simulink subsystem "EvPowertrainController2EM_r3"  (R2025b)
settings: Solver=VariableStepAuto  StartTime=0.0  StopTime=10.0  RelTol=1e-3
undefined symbols (not defined in the file): CtrlVcuAccelPdlBpts, CtrlVcuBattPnlty, CtrlVcuEMPnlty, CtrlVcuEMTrqSplitGrid, CtrlVcuEvChrgLmtBpt, CtrlVcuEvRegenBrkCutOff, CtrlVcuEvRegenBrkSpdBpt, CtrlVcuEvSocBpt, CtrlVcuFallRate, CtrlVcuMaxAccelG, CtrlVcuMaxDecelG, CtrlVcuPwrRatePnlty, CtrlVcuRiseRate, CtrlVcuRoadMuEst, CtrlVcuSftyFctr, CtrlVcuTracPwrErrPnlty, DriverMode, eff, EnvGrvty, PlntBrkActrBoreFrnt, PlntBrkFrntBias, PlntBrkKinFricCffFrnt, PlntBrkNumPadsFrnt, PlntBrkPadMeanRadiusFrnt, PlntBrkPrsFctr, PlntBrkRearBias, PlntDiffrntl2Eff, PlntDiffrntl2Ratio, PlntDiffrntlEff, PlntDiffrntlRatio, PlntEM1EffTbl, PlntEM1Spd, PlntEM1Trq, PlntEM1TrqEff, PlntEM2EffTbl, PlntEM2Spd, PlntEM2Trq, PlntEM2TrqEff, PlntEM3EffTbl, PlntEM3Spd, PlntEM3Trq, PlntEM3TrqEff, PlntEMWhlGearEffFL, PlntEMWhlGearEffRL, PlntEMWhlGearRatioFL, PlntEMWhlGearRatioRL, PlntTransEffSpdBpt, PlntTransEffTbl, PlntTransEffTempBpt, PlntTransEffTrqBpt, PlntTransGearNumVect, PlntTransGearRatioVect, PlntVehCGHgtAxl, PlntVehDstCGFrntAxl, PlntVehDstCGRearAxl, PlntVehMass, PlntWhlLdRadius, RegenEnd, RegenStrt, SOCInit ... (+1)
libraries: simulink x13, autolibutils x2
(part 1 of 5)
settings Model: Creator=smuckati  LastModifiedBy=smuckati
settings RTWCC: GPUComputeCapability=3.5

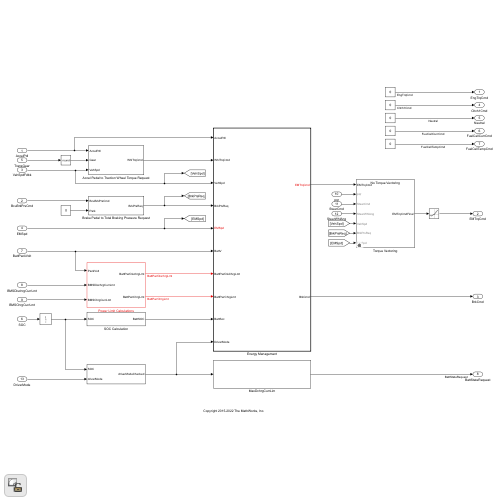
[thumbnail: Simulink's stored preview of the top-level diagram]
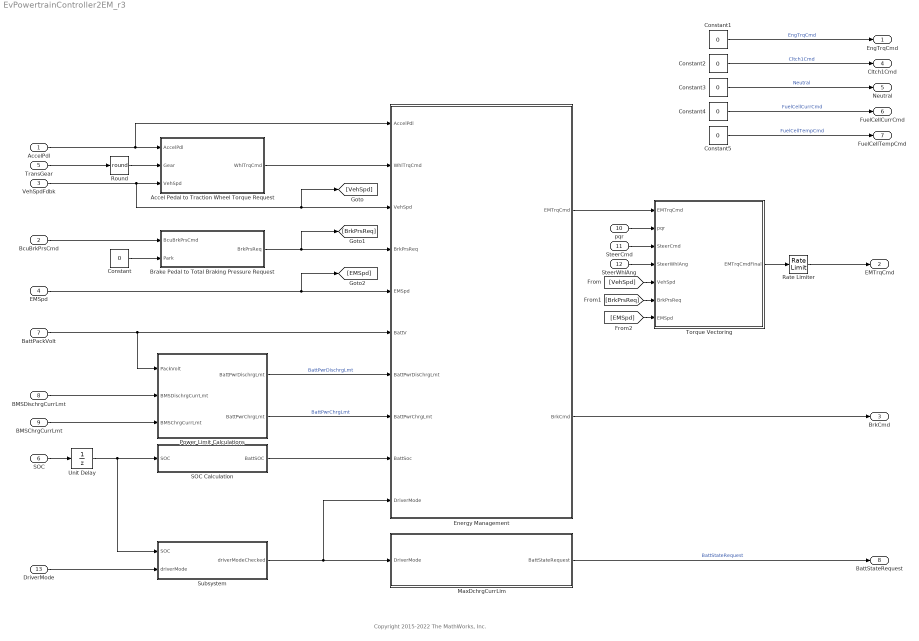
== system EvPowertrainController2EM_r3 ==
  note: Copyright 2015-2022 The MathWorks, Inc.
  AccelPdl : Inport
  BcuBrkPrsCmd : Inport  Port=2  PortDimensions=4
  VehSpdFdbk : Inport  Port=3
  EMSpd : Inport  Port=4
  TransGear : Inport  Port=5
  SOC : Inport  Port=6
  BattPackVolt : Inport  Port=7
  BMSDischrgCurrLmt : Inport  Port=8
  BMSChrgCurrLmt : Inport  Port=9
  pqr : Inport  Port=10  PortDimensions=3
  SteerCmd : Inport  Port=11
  SteerWhlAng : Inport  Port=12  PortDimensions=4
  DriverMode : Inport  Port=13
  Accel Pedal to Traction Wheel Torque Request : Subsystem  InitFcn=[~]=autosharedicon('autolibinternalvvblock',gcb,0);  VariantControl=Choice
  Brake Pedal to Total Braking Pressure Request : Subsystem  InitFcn=[~]=autosharedicon('autolibinternalvvblock',gcb,0);
  Constant{,1..5} (6 alike) : Constant  Value=0  SampleTime=-1
  Energy Management : Subsystem  LoadFcn=[~]=autosharedicon('autolibinternalvvblock',gcb,0);  TreatAsAtomicUnit=on
  MaxDchrgCurrLim : Subsystem
  Power Limit Calculations : Subsystem  InitFcn=[~]=autosharedicon('autolibinternalvvblock',gcb,0);
  Rate Limiter : RateLimiter  RisingSlewLimit=CtrlVcuRiseRate  FallingSlewLimit=CtrlVcuFallRate  SampleTimeMode=inherited
  Round : Rounding  Operator=round
  SOC Calculation : Subsystem  InitFcn=[~]=autosharedicon('autolibinternalvvblock',gcb,0);
  Subsystem : Subsystem
  Torque Vectoring : Subsystem  Variant=on  VariantControlMode=label  VariantControl=Choice  LabelModeActiveChoice=No Torque Vectoring
  Unit Delay : UnitDelay  InitialCondition=SOCInit  SampleTime=-1  HasFrameUpgradeWarning=on
  EngTrqCmd : Outport
  EMTrqCmd : Outport  Port=2
  BrkCmd : Outport  Port=3
  Cltch1Cmd : Outport  Port=4
  Neutral : Outport  Port=5
  FuelCellCurrCmd : Outport  Port=6
  FuelCellTempCmd : Outport  Port=7
  BattStateRequest : Outport  Port=8
  wires:
  Rate Limiter/1 -> EMTrqCmd/1
  AccelPdl/1 -> Accel Pedal to Traction Wheel Torque Request/1(AccelPdl), Energy Management/1(AccelPdl)
  Constant/1 -> Brake Pedal to Total Braking Pressure Request/2(Park)
  EMSpd/1 -> Energy Management/5(EMSpd), [EMSpd]
  Power Limit Calculations/2(BattPwrChrgLmt) -> Energy Management/8("BattPwrChrgLmt ")  "BattPwrChrgLmt"
  [BrkPrsReq] -> Torque Vectoring/6(BrkPrsReq)
  Accel Pedal to Traction Wheel Torque Request/1(WhlTrqCmd) -> Energy Management/2(WhlTrqCmd)
  BattPackVolt/1 -> Power Limit Calculations/1(PackVolt), Energy Management/6(BattV)
  Brake Pedal to Total Braking Pressure Request/1(BrkPrsReq) -> Energy Management/4("BrkPrsReq "), [BrkPrsReq]
  SOC Calculation/1(BattSOC) -> Energy Management/9(BattSoc)
  BcuBrkPrsCmd/1 -> Brake Pedal to Total Braking Pressure Request/1(BcuBrkPrsCmd)
  pqr/1 -> Torque Vectoring/2(pqr)
  [VehSpd] -> Torque Vectoring/5(VehSpd)
  VehSpdFdbk/1 -> Accel Pedal to Traction Wheel Torque Request/3(VehSpd), Energy Management/3(VehSpd), [VehSpd]
  SteerCmd/1 -> Torque Vectoring/3(SteerCmd)
  SteerWhlAng/1 -> Torque Vectoring/4(SteerWhlAng)
  Round/1 -> Accel Pedal to Traction Wheel Torque Request/2(Gear)
  Energy Management/2(BrkCmd) -> BrkCmd/1
  Energy Management/1(EMTrqCmd) -> Torque Vectoring/1(EMTrqCmd)
  [EMSpd] -> Torque Vectoring/7(EMSpd)
  Power Limit Calculations/1(BattPwrDischrgLmt) -> Energy Management/7(BattPwrDisChrgLmt)  "BattPwrDischrgLmt"
  Torque Vectoring/1(EMTrqCmdFinal) -> Rate Limiter/1
  Constant5/1 -> FuelCellTempCmd/1  "FuelCellTempCmd"
  MaxDchrgCurrLim/1(BattStateRequest) -> BattStateRequest/1  "BattStateRequest"
  SOC/1 -> Unit Delay/1
  TransGear/1 -> Round/1
  Constant4/1 -> FuelCellCurrCmd/1  "FuelCellCurrCmd"
  Constant2/1 -> Cltch1Cmd/1  "Cltch1Cmd"
  BMSDischrgCurrLmt/1 -> Power Limit Calculations/2(BMSDischrgCurrLmt)
  Constant1/1 -> EngTrqCmd/1  "EngTrqCmd"
  Constant3/1 -> Neutral/1  "Neutral"
  BMSChrgCurrLmt/1 -> Power Limit Calculations/3(BMSChrgCurrLmt)
  DriverMode/1 -> Subsystem/2(driverMode)
  Subsystem/1(driverModeChecked) -> MaxDchrgCurrLim/1(DriverMode), Energy Management/10(DriverMode)
  Unit Delay/1 -> SOC Calculation/1(SOC), Subsystem/1(SOC)

== system EvPowertrainController2EM_r3/Accel Pedal to Traction Wheel Torque Request ==
  note: Convert Accelerator Pedal Position to
      | Wheel Torque Command using Motor
      | Torque Speed Curves.
      |
      | Can be replaced with 2D Lookup Table
      | with AccelPdl and VehSpd as inputs and
      | Motor or Wheel Torque Command as output.
  AccelPdl : Inport
  Gear : Inport  Port=2
  VehSpd : Inport  Port=3
  EM2WhlTrq : Subsystem  Variant=on  VariantControlMode=label  VariantControl=Choice  LabelModeActiveChoice=2EM
  Product1 : Product
  WhlTrqCmd : Outport  VectorParamsAs1DForOutWhenUnconnected=off
  wires:
  EM2WhlTrq/1(WhlTrqCmd) -> Product1/2
  VehSpd/1 -> EM2WhlTrq/2(VehSpd)
  Gear/1 -> EM2WhlTrq/1(Gear)
  AccelPdl/1 -> Product1/1
  Product1/1 -> WhlTrqCmd/1

== system EvPowertrainController2EM_r3/Brake Pedal to Total Braking Pressure Request ==
  BcuBrkPrsCmd : Inport
  Park : Inport  Port=2
  Front Bias : Constant  Value=PlntBrkFrntBias
  Gain4 : Gain  Gain=PlntBrkPrsFctr
  Mux : Mux
  Product : Product
  Rear Bias : Constant  Value=PlntBrkRearBias
  Terminator : Terminator
  BrkPrsReq : Outport  VectorParamsAs1DForOutWhenUnconnected=off
  wires:
  Park/1 -> Terminator/1
  Product/1 -> Gain4/1
  Gain4/1 -> BrkPrsReq/1
  Front Bias/1 -> Mux/2, Mux/1
  Rear Bias/1 -> Mux/3, Mux/4
  Mux/1 -> Product/1
  BcuBrkPrsCmd/1 -> Product/2

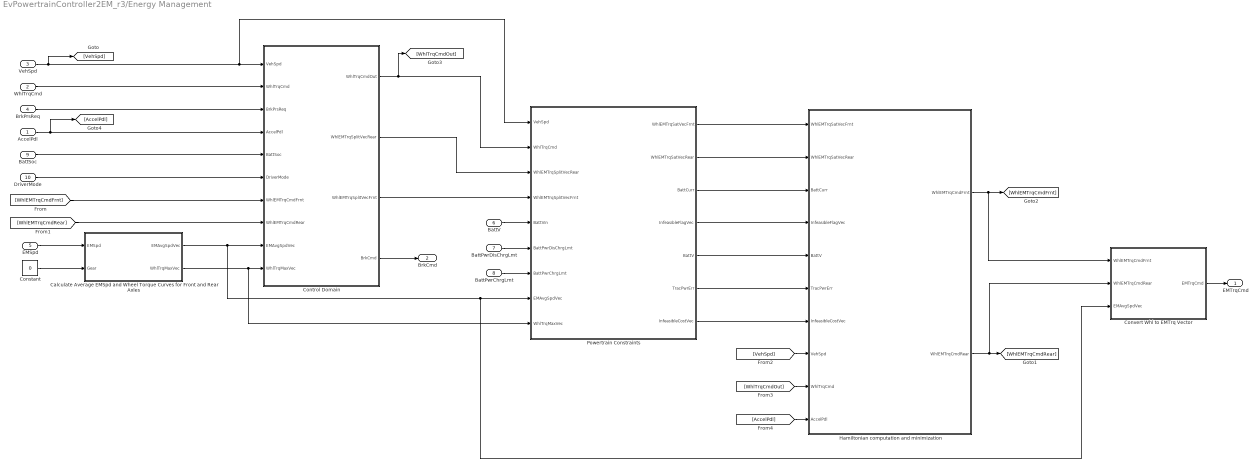
== system EvPowertrainController2EM_r3/Energy Management ==
  AccelPdl : Inport
  WhlTrqCmd : Inport  Port=2
  VehSpd : Inport  Port=3
  "BrkPrsReq " : Inport  Port=4
  EMSpd : Inport  Port=5
  BattV : Inport  Port=6
  BattPwrDisChrgLmt : Inport  Port=7
  "BattPwrChrgLmt " : Inport  Port=8
  BattSoc : Inport  Port=9
  DriverMode : Inport  Port=10
  Calculate Average EMSpd and Wheel Torque Curves for Front and Rear Axles : Subsystem  Variant=on  VariantControlMode=label  VariantControl=Choice  LabelModeActiveChoice=2EM
  Constant : Constant  Value=0  SampleTime=-1
  "Control Domain " : Subsystem  InitFcn="[~] =  autosharedeval('1');"
  Convert Whl to EMTrq Vector : Subsystem  Variant=on  VariantControlMode=label  VariantControl=Choice  LabelModeActiveChoice=2EM
  Hamiltonian computation and minimization : Subsystem  InitFcn="[~] =  autosharedeval('1');"
  "Powertrain Constraints " : Subsystem  InitFcn="[~] =  autosharedeval('1');"
  EMTrqCmd : Outport  VectorParamsAs1DForOutWhenUnconnected=off
  BrkCmd : Outport  Port=2  VectorParamsAs1DForOutWhenUnconnected=off
  wires:
  DriverMode/1 -> "Control Domain "/6(DriverMode)
  [AccelPdl] -> Hamiltonian computation and minimization/10(AccelPdl)
  [WhlTrqCmdOut] -> Hamiltonian computation and minimization/9(WhlTrqCmd)
  "Control Domain "/3(WhlEMTrqSplitVecFrnt) -> "Powertrain Constraints "/4(WhlEMTrqSplitVecFrnt)
  "Powertrain Constraints "/7(InfeasibleCostVec) -> Hamiltonian computation and minimization/7(InfeasibleCostVec)
  [VehSpd] -> Hamiltonian computation and minimization/8(VehSpd)
  "Powertrain Constraints "/2(WhlEMTrqSatVecRear) -> Hamiltonian computation and minimization/2(WhlEMTrqSatVecRear)
  "Powertrain Constraints "/1(WhlEMTrqSatVecFrnt) -> Hamiltonian computation and minimization/1(WhlEMTrqSatVecFrnt)
  Calculate Average EMSpd and Wheel Torque Curves for Front and Rear Axles/2(WhlTrqMaxVec) -> "Control Domain "/10(WhlTrqMaxVec), "Powertrain Constraints "/9(WhlTrqMaxVec)
  Constant/1 -> Calculate Average EMSpd and Wheel Torque Curves for Front and Rear Axles/2(Gear)
  [WhlEMTrqCmdRear] -> "Control Domain "/8(WhlEMTrqCmdRear)
  Convert Whl to EMTrq Vector/1(EMTrqCmd) -> EMTrqCmd/1
  EMSpd/1 -> Calculate Average EMSpd and Wheel Torque Curves for Front and Rear Axles/1(EMSpd)
  BattSoc/1 -> "Control Domain "/5(BattSoc)
  [WhlEMTrqCmdFrnt] -> "Control Domain "/7(WhlEMTrqCmdFrnt)
  BattPwrDisChrgLmt/1 -> "Powertrain Constraints "/6(BattPwrDisChrgLmt)
  "BattPwrChrgLmt "/1 -> "Powertrain Constraints "/7("BattPwrChrgLmt ")
  Calculate Average EMSpd and Wheel Torque Curves for Front and Rear Axles/1(EMAvgSpdVec) -> "Control Domain "/9(EMAvgSpdVec), "Powertrain Constraints "/8(EMAvgSpdVec), Convert Whl to EMTrq Vector/3(EMAvgSpdVec)
  "Control Domain "/2(WhlEMTrqSplitVecRear) -> "Powertrain Constraints "/3(WhlEMTrqSplitVecRear)
  WhlTrqCmd/1 -> "Control Domain "/2(WhlTrqCmd)
  "Powertrain Constraints "/5(BattV) -> Hamiltonian computation and minimization/5(BattV)
  "Powertrain Constraints "/3(BattCurr) -> Hamiltonian computation and minimization/3(BattCurr)
  "Powertrain Constraints "/4(InfeasibleFlagVec) -> Hamiltonian computation and minimization/4(InfeasibleFlagVec)
  Hamiltonian computation and minimization/1(WhlEMTrqCmdFrnt) -> [WhlEMTrqCmdFrnt], Convert Whl to EMTrq Vector/1(WhlEMTrqCmdFrnt)
  Hamiltonian computation and minimization/2(WhlEMTrqCmdRear) -> [WhlEMTrqCmdRear], Convert Whl to EMTrq Vector/2(WhlEMTrqCmdRear)
  VehSpd/1 -> "Control Domain "/1(VehSpd), "Powertrain Constraints "/1(VehSpd), [VehSpd]
  BattV/1 -> "Powertrain Constraints "/5(BattVin)
  "Powertrain Constraints "/6(TracPwrErr) -> Hamiltonian computation and minimization/6(TracPwrErr)
  "Control Domain "/4(BrkCmd) -> BrkCmd/1
  AccelPdl/1 -> [AccelPdl], "Control Domain "/4(AccelPdl)
  "BrkPrsReq "/1 -> "Control Domain "/3("BrkPrsReq ")
  "Control Domain "/1(WhlTrqCmdOut) -> "Powertrain Constraints "/2(WhlTrqCmd), [WhlTrqCmdOut]

== system EvPowertrainController2EM_r3/MaxDchrgCurrLim ==
  note: Setup Battery Operating Mode
  DriverMode : Inport
  Cast To Double : DataTypeConversion  OutDataTypeStr=int8  SaturateOnIntegerOverflow=off  RndMeth=Floor
  Enumerated Constant : simulink/Sources/Enumerated Constant  OutDataTypeStr=Enum: SRE  Value=SRE.SportMode  SampleTime=inf
  Enumerated Constant1 : simulink/Sources/Enumerated Constant  OutDataTypeStr=Enum: SRE  Value=SRE.Driving  SampleTime=inf
  Switch : Switch  Threshold=1  SaturateOnIntegerOverflow=off  InputSameDT=off
  BattStateRequest : Outport
  wires:
  Switch/1 -> BattStateRequest/1
  Cast To Double/1 -> Switch/2
  DriverMode/1 -> Cast To Double/1
  Enumerated Constant/1 -> Switch/1
  Enumerated Constant1/1 -> Switch/3

== system EvPowertrainController2EM_r3/Power Limit Calculations ==
  note: Use Current Limits from BMS to calculate
      | discharge and charge power limits
  note: BMS has opposite sign convention for current
  PackVolt : Inport
  BMSDischrgCurrLmt : Inport  Port=2
  BMSChrgCurrLmt : Inport  Port=3
  Data Type Conversion : DataTypeConversion  SaturateOnIntegerOverflow=off  RndMeth=Floor
  Data Type Conversion1 : DataTypeConversion  SaturateOnIntegerOverflow=off  RndMeth=Floor
  Gain : Gain  Gain=-1
  Gain1 : Gain  Gain=-1
  Product : Product
  Product1 : Product
  BattPwrDischrgLmt : Outport  VectorParamsAs1DForOutWhenUnconnected=off
  BattPwrChrgLmt : Outport  Port=2  VectorParamsAs1DForOutWhenUnconnected=off
  wires:
  Data Type Conversion1/1 -> BattPwrDischrgLmt/1
  Data Type Conversion/1 -> BattPwrChrgLmt/1
  BMSDischrgCurrLmt/1 -> Gain1/1
  BMSChrgCurrLmt/1 -> Gain/1
  PackVolt/1 -> Product1/1, Product/1
  Product1/1 -> Data Type Conversion/1
  Product/1 -> Data Type Conversion1/1
  Gain1/1 -> Product/2
  Gain/1 -> Product1/2

== system EvPowertrainController2EM_r3/SOC Calculation ==
  SOC : Inport
  Data Type Conversion : DataTypeConversion  SaturateOnIntegerOverflow=off  RndMeth=Floor
  convert2percent : Gain  Gain=100
  BattSOC : Outport
  wires:
  Data Type Conversion/1 -> BattSOC/1
  SOC/1 -> convert2percent/1
  convert2percent/1 -> Data Type Conversion/1

== system EvPowertrainController2EM_r3/Subsystem ==
  SOC : Inport
  driverMode : Inport  Port=2
  Enumerated Constant : simulink/Sources/Enumerated Constant  OutDataTypeStr=Enum: DriverMode  Value=DriverMode.Comfort  SampleTime=inf
  Switch : Switch  Threshold=0.25  SaturateOnIntegerOverflow=off  InputSameDT=off
  driverModeChecked : Outport
  wires:
  Enumerated Constant/1 -> Switch/3
  driverMode/1 -> Switch/1
  Switch/1 -> driverModeChecked/1
  SOC/1 -> Switch/2

== system EvPowertrainController2EM_r3/Torque Vectoring ==
  EMTrqCmd : Inport
  pqr : Inport  Port=2
  SteerCmd : Inport  Port=3
  SteerWhlAng : Inport  Port=4
  VehSpd : Inport  Port=5
  BrkPrsReq : Inport  Port=6
  EMSpd : Inport  Port=7
  No Torque Vectoring : Subsystem  VariantControl=No Torque Vectoring
  EMTrqCmdFinal : Outport

== system EvPowertrainController2EM_r3/Accel Pedal to Traction Wheel Torque Request/EM2WhlTrq ==
  Gear : Inport
  VehSpd : Inport  Port=2
  2EM : Subsystem  VariantControl=2EM
  3EM Dual Front : Subsystem  VariantControl=3EM Dual Front
  3EM Dual Rear : Subsystem  VariantControl=3EM Dual Rear
  4EM : Subsystem  VariantControl=4EM
  WhlTrqCmd : Outport

== system EvPowertrainController2EM_r3/Energy Management/Calculate Average EMSpd and Wheel Torque Curves for Front and Rear Axles ==
  EMSpd : Inport
  Gear : Inport  Port=2
  2EM : Subsystem  VariantControl=2EM
  3EM Dual Front : Subsystem  VariantControl=3EM Dual Front
  3EM Dual Rear : Subsystem  VariantControl=3EM Dual Rear
  4EM : Subsystem  VariantControl=4EM
  EMAvgSpdVec : Outport
  WhlTrqMaxVec : Outport  Port=2

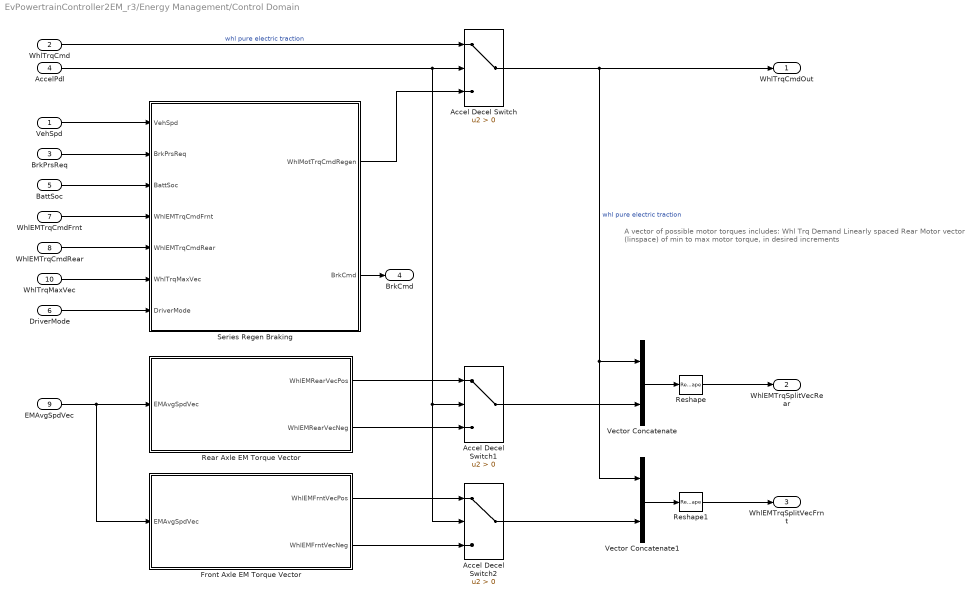
== system EvPowertrainController2EM_r3/Energy Management/Control Domain  ==
  note: A vector of possible motor torques includes:
      | Whl Trq Demand
      | Linearly spaced Rear Motor vector (linspace) of min to max motor torque, in desired increments
  VehSpd : Inport
  WhlTrqCmd : Inport  Port=2
  "BrkPrsReq " : Inport  Port=3
  AccelPdl : Inport  Port=4
  BattSoc : Inport  Port=5
  DriverMode : Inport  Port=6
  WhlEMTrqCmdFrnt : Inport  Port=7
  WhlEMTrqCmdRear : Inport  Port=8
  EMAvgSpdVec : Inport  Port=9
  WhlTrqMaxVec : Inport  Port=10
  Accel Decel Switch : Switch  Criteria=u2 > Threshold  SaturateOnIntegerOverflow=off  InputSameDT=off
  Accel Decel Switch1 : Switch  Criteria=u2 > Threshold  SaturateOnIntegerOverflow=off  InputSameDT=off
  Accel Decel Switch2 : Switch  Criteria=u2 > Threshold  SaturateOnIntegerOverflow=off  InputSameDT=off
  Front Axle EM Torque Vector : Subsystem  Variant=on  VariantControlMode=label  VariantControl=Choice  LabelModeActiveChoice=2EM or 3EM Dual Rear
  Rear Axle EM Torque Vector : Subsystem  Variant=on  VariantControlMode=label  VariantControl=Choice  LabelModeActiveChoice=2EM or 3EM Dual Front
  Reshape : Reshape
  Reshape1 : Reshape
  Series Regen Braking : Subsystem  InitFcn=%[~]=autosharedicon('autolibutils',gcb,0);  VariantControl=Variant
  Vector Concatenate : Concatenate
  Vector Concatenate1 : Concatenate
  WhlTrqCmdOut : Outport  VectorParamsAs1DForOutWhenUnconnected=off
  WhlEMTrqSplitVecRear : Outport  Port=2  VectorParamsAs1DForOutWhenUnconnected=off
  WhlEMTrqSplitVecFrnt : Outport  Port=3  VectorParamsAs1DForOutWhenUnconnected=off
  BrkCmd : Outport  Port=4  VectorParamsAs1DForOutWhenUnconnected=off
  wires:
  DriverMode/1 -> Series Regen Braking/7(DriverMode)
  Accel Decel Switch2/1 -> Vector Concatenate1/2
  Front Axle EM Torque Vector/2(WhlEMFrntVecNeg) -> Accel Decel Switch2/3
  Front Axle EM Torque Vector/1(WhlEMFrntVecPos) -> Accel Decel Switch2/1
  Vector Concatenate1/1 -> Reshape1/1
  Reshape1/1 -> WhlEMTrqSplitVecFrnt/1
  Rear Axle EM Torque Vector/2(WhlEMRearVecNeg) -> Accel Decel Switch1/3
  Rear Axle EM Torque Vector/1(WhlEMRearVecPos) -> Accel Decel Switch1/1
  BattSoc/1 -> Series Regen Braking/3(BattSoc)
  WhlEMTrqCmdRear/1 -> Series Regen Braking/5(WhlEMTrqCmdRear)
  WhlEMTrqCmdFrnt/1 -> Series Regen Braking/4(WhlEMTrqCmdFrnt)
  Series Regen Braking/1(" WhlMotTrqCmdRegen") -> Accel Decel Switch/3
  Accel Decel Switch1/1 -> Vector Concatenate/2
  Accel Decel Switch/1 -> WhlTrqCmdOut/1, Vector Concatenate1/1, Vector Concatenate/1  "whl pure electric traction"
  VehSpd/1 -> Series Regen Braking/1(VehSpd)
  EMAvgSpdVec/1 -> Rear Axle EM Torque Vector/1(EMAvgSpdVec), Front Axle EM Torque Vector/1(EMAvgSpdVec)
  "BrkPrsReq "/1 -> Series Regen Braking/2("BrkPrsReq ")
  WhlTrqCmd/1 -> Accel Decel Switch/1  "whl pure electric traction"
  Series Regen Braking/2(" BrkCmd") -> BrkCmd/1
  AccelPdl/1 -> Accel Decel Switch/2, Accel Decel Switch1/2, Accel Decel Switch2/2
  WhlTrqMaxVec/1 -> Series Regen Braking/6(WhlTrqMaxVec)
  Reshape/1 -> WhlEMTrqSplitVecRear/1
  Vector Concatenate/1 -> Reshape/1

== system EvPowertrainController2EM_r3/Energy Management/Convert Whl to EMTrq Vector ==
  WhlEMTrqCmdFrnt : Inport
  WhlEMTrqCmdRear : Inport  Port=2
  EMAvgSpdVec : Inport  Port=3
  2EM : Subsystem  VariantControl=2EM
  3EM Dual Front : Subsystem  VariantControl=3EM Dual Front
  3EM Dual Rear : Subsystem  VariantControl=3EM Dual Rear
  4EM : Subsystem  VariantControl=4EM
  EMTrqCmd : Outport

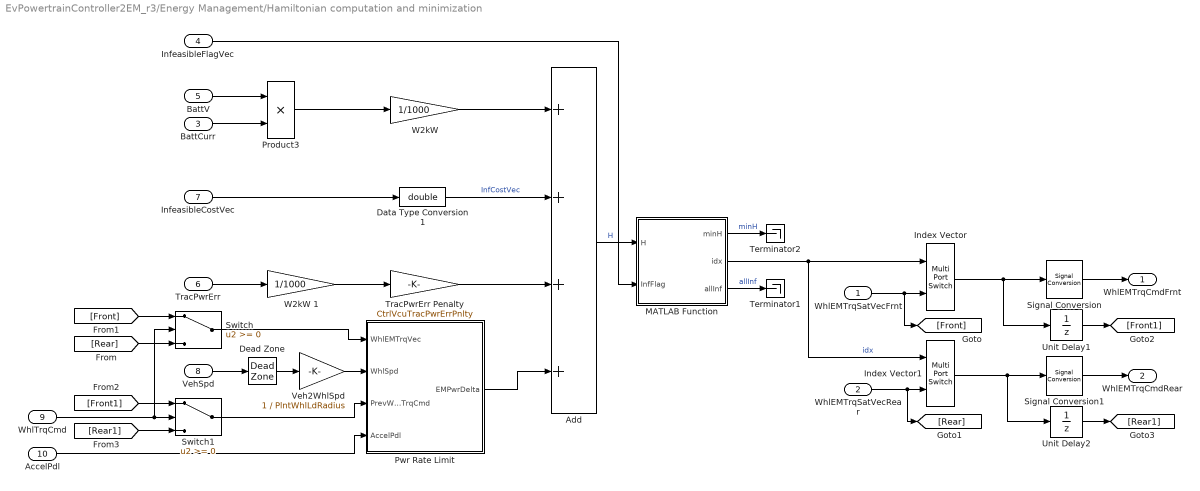
== system EvPowertrainController2EM_r3/Energy Management/Hamiltonian computation and minimization ==
  WhlEMTrqSatVecFrnt : Inport
  WhlEMTrqSatVecRear : Inport  Port=2
  BattCurr : Inport  Port=3
  InfeasibleFlagVec : Inport  Port=4
  BattV : Inport  Port=5
  TracPwrErr : Inport  Port=6
  InfeasibleCostVec : Inport  Port=7
  VehSpd : Inport  Port=8
  WhlTrqCmd : Inport  Port=9
  AccelPdl : Inport  Port=10
  Add : Sum  Inputs=++++
  Data Type Conversion1 : DataTypeConversion  OutDataTypeStr=double  SaturateOnIntegerOverflow=off  RndMeth=Floor
  Dead Zone : DeadZone  LowerValue=-0.1  UpperValue=0.1
  Index Vector : MultiPortSwitch  Inputs=1  SaturateOnIntegerOverflow=off  InputSameDT=off
  Index Vector1 : MultiPortSwitch  Inputs=1  SaturateOnIntegerOverflow=off  InputSameDT=off
  MATLAB Function : MATLAB Function  InitFcn="[~] =  autosharedeval('1');"  TreatAsAtomicUnit=on
  Product3 : Product
  Pwr Rate Limit : Subsystem  InitFcn="[~] =  autosharedeval('1');"
  Signal Conversion : SignalConversion  OverrideOpt=off
  Signal Conversion1 : SignalConversion  OverrideOpt=off
  Switch : Switch  SaturateOnIntegerOverflow=off  InputSameDT=off
  Switch1 : Switch  SaturateOnIntegerOverflow=off  InputSameDT=off
  Terminator1 : Terminator
  Terminator2 : Terminator
  TracPwrErr Penalty : Gain  Gain=CtrlVcuTracPwrErrPnlty
  Unit Delay1 : UnitDelay  SampleTime=-1  HasFrameUpgradeWarning=on
  Unit Delay2 : UnitDelay  SampleTime=-1  HasFrameUpgradeWarning=on
  Veh2WhlSpd : Gain  Gain=1 / PlntWhlLdRadius
  "W2kW " : Gain  Gain=1/1000
  W2kW 1 : Gain  Gain=1/1000
  WhlEMTrqCmdFrnt : Outport  VectorParamsAs1DForOutWhenUnconnected=off
  WhlEMTrqCmdRear : Outport  Port=2  VectorParamsAs1DForOutWhenUnconnected=off
  wires:
  AccelPdl/1 -> Pwr Rate Limit/4(AccelPdl)
  Switch1/1 -> Pwr Rate Limit/3(PrevWhlEMTrqCmd)
  Switch/1 -> Pwr Rate Limit/1(WhlEMTrqVec)
  Dead Zone/1 -> Veh2WhlSpd/1
  [Rear1] -> Switch1/3
  Unit Delay2/1 -> [Rear1]
  Unit Delay1/1 -> [Front1]
  WhlTrqCmd/1 -> Switch1/2, Switch/2
  BattCurr/1 -> Product3/2
  [Front1] -> Switch1/1
  [Rear] -> Switch/3
  InfeasibleCostVec/1 -> Data Type Conversion1/1
  VehSpd/1 -> Dead Zone/1
  Pwr Rate Limit/1(EMPwrDelta) -> Add/4
  MATLAB Function/3(allInf) -> Terminator1/1  "allInf"
  Veh2WhlSpd/1 -> Pwr Rate Limit/2(WhlSpd)
  [Front] -> Switch/1
  Product3/1 -> "W2kW "/1
  WhlEMTrqSatVecFrnt/1 -> Index Vector/2, [Front]
  InfeasibleFlagVec/1 -> MATLAB Function/2(InfFlag)
  WhlEMTrqSatVecRear/1 -> Index Vector1/2, [Rear]
  MATLAB Function/2(idx) -> Index Vector/1, Index Vector1/1  "idx"
  MATLAB Function/1(minH) -> Terminator2/1  "minH"
  Add/1 -> MATLAB Function/1(H)  "H"
  Index Vector1/1 -> Signal Conversion1/1, Unit Delay2/1
  BattV/1 -> Product3/1
  "W2kW "/1 -> Add/1
  Index Vector/1 -> Signal Conversion/1, Unit Delay1/1
  Signal Conversion/1 -> WhlEMTrqCmdFrnt/1
  Signal Conversion1/1 -> WhlEMTrqCmdRear/1
  TracPwrErr/1 -> W2kW 1/1
  W2kW 1/1 -> TracPwrErr Penalty/1
  TracPwrErr Penalty/1 -> Add/3
  Data Type Conversion1/1 -> Add/2  "InfCostVec"

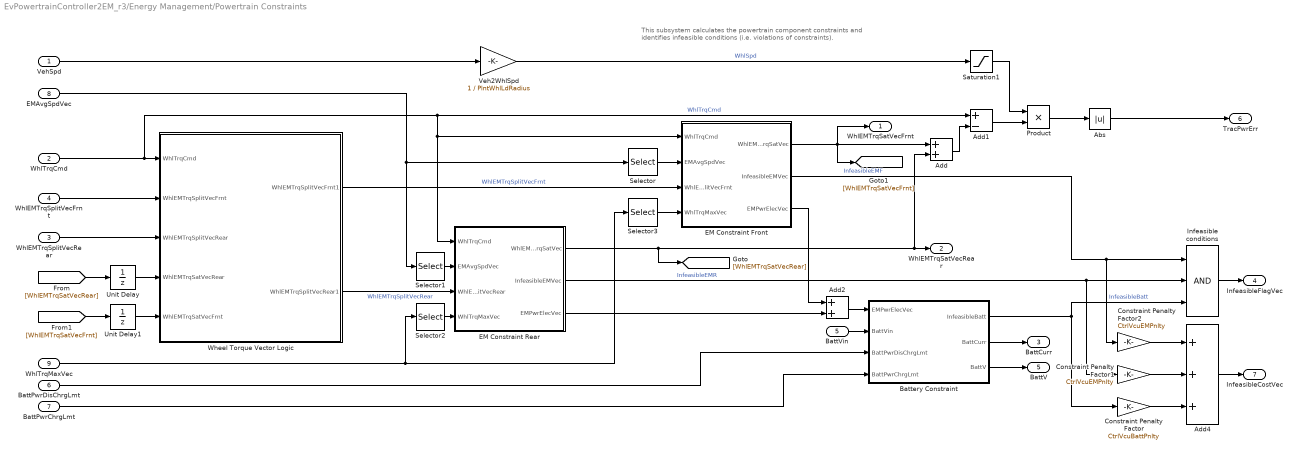
== system EvPowertrainController2EM_r3/Energy Management/Powertrain Constraints  ==
  note: This subsystem calculates the powertrain component constraints
      | and identifies infeasible conditions (i.e. violations of constraints).
  VehSpd : Inport
  WhlTrqCmd : Inport  Port=2
  WhlEMTrqSplitVecRear : Inport  Port=3
  WhlEMTrqSplitVecFrnt : Inport  Port=4
  BattVin : Inport  Port=5
  BattPwrDisChrgLmt : Inport  Port=6
  "BattPwrChrgLmt " : Inport  Port=7
  EMAvgSpdVec : Inport  Port=8
  WhlTrqMaxVec : Inport  Port=9
  Abs : Abs  SaturateOnIntegerOverflow=off
  Add : Sum
  Add1 : Sum  Inputs=+-
  Add2 : Sum
  Add4 : Sum  Inputs=+++
  Battery Constraint : Subsystem  InitFcn="[~] =  autosharedeval('1');"
  Constraint Penalty Factor : Gain  Gain=CtrlVcuBattPnlty
  Constraint Penalty Factor1 : Gain  Gain=CtrlVcuEMPnlty
  Constraint Penalty Factor2 : Gain  Gain=CtrlVcuEMPnlty
  EM Constraint Front : Subsystem  InitFcn="[~] =  autosharedeval('1');"
  EM Constraint Rear : Subsystem  InitFcn="[~] =  autosharedeval('1');"
  Infeasible conditions : Logic  Inputs=3  AllPortsSameDT=off  OutDataTypeStr=boolean
  Product : Product
  Saturation1 : Saturate  UpperLimit=inf  LowerLimit=0.001
  Selector : Selector  InputPortWidth=2  IndexOptions=Index vector (dialog)  Indices=[1]  OutputSizes=1
  Selector1 : Selector  InputPortWidth=2  IndexOptions=Index vector (dialog)  Indices=[2]  OutputSizes=1
  Selector2 : Selector  InputPortWidth=2  IndexOptions=Index vector (dialog)  Indices=[2]  OutputSizes=1
  Selector3 : Selector  InputPortWidth=2  IndexOptions=Index vector (dialog)  Indices=[1]  OutputSizes=1
  Unit Delay : UnitDelay  SampleTime=-1  HasFrameUpgradeWarning=on
  Unit Delay1 : UnitDelay  SampleTime=-1  HasFrameUpgradeWarning=on
  Veh2WhlSpd : Gain  Gain=1 / PlntWhlLdRadius
  Wheel Torque Vector Logic : Subsystem
  WhlEMTrqSatVecFrnt : Outport  VectorParamsAs1DForOutWhenUnconnected=off
  WhlEMTrqSatVecRear : Outport  Port=2  VectorParamsAs1DForOutWhenUnconnected=off
  BattCurr : Outport  Port=3  VectorParamsAs1DForOutWhenUnconnected=off
  InfeasibleFlagVec : Outport  Port=4  VectorParamsAs1DForOutWhenUnconnected=off
  BattV : Outport  Port=5  VectorParamsAs1DForOutWhenUnconnected=off
  TracPwrErr : Outport  Port=6  VectorParamsAs1DForOutWhenUnconnected=off
  InfeasibleCostVec : Outport  Port=7  VectorParamsAs1DForOutWhenUnconnected=off
  wires:
  Unit Delay1/1 -> Wheel Torque Vector Logic/5(WhlEMTrqSatVecFrnt)
  Unit Delay/1 -> Wheel Torque Vector Logic/4(WhlEMTrqSatVecRear)
  [WhlEMTrqSatVecFrnt] -> Unit Delay1/1
  [WhlEMTrqSatVecRear] -> Unit Delay/1
  Wheel Torque Vector Logic/2(WhlEMTrqSplitVecRear1) -> EM Constraint Rear/3(WhlEMTrqSplitVecRear)  "WhlEMTrqSplitVecRear"
  WhlEMTrqSplitVecRear/1 -> Wheel Torque Vector Logic/3(WhlEMTrqSplitVecRear)
  WhlEMTrqSplitVecFrnt/1 -> Wheel Torque Vector Logic/2(WhlEMTrqSplitVecFrnt)
  WhlTrqMaxVec/1 -> Selector3/1, Selector2/1
  VehSpd/1 -> Veh2WhlSpd/1
  "BattPwrChrgLmt "/1 -> Battery Constraint/4("BattPwrChrgLmt ")
  BattPwrDisChrgLmt/1 -> Battery Constraint/3(BattPwrDisChrgLmt)
  Constraint Penalty Factor2/1 -> Add4/1
  Constraint Penalty Factor1/1 -> Add4/2
  Constraint Penalty Factor/1 -> Add4/3
  Add4/1 -> InfeasibleCostVec/1
  Selector3/1 -> EM Constraint Front/4(WhlTrqMaxVec)
  Selector2/1 -> EM Constraint Rear/4(WhlTrqMaxVec)
  Selector1/1 -> EM Constraint Rear/2(EMAvgSpdVec)
  Selector/1 -> EM Constraint Front/2(EMAvgSpdVec)
  EM Constraint Front/3(EMPwrElecVec) -> Add2/1
  Product/1 -> Abs/1
  Wheel Torque Vector Logic/1(WhlEMTrqSplitVecFrnt1) -> EM Constraint Front/3(WhlEMTrqSplitVecFrnt)  "WhlEMTrqSplitVecFrnt"
  EMAvgSpdVec/1 -> Selector1/1, Selector/1
  Battery Constraint/3(BattV) -> BattV/1
  EM Constraint Rear/3(EMPwrElecVec) -> Add2/2
  Add2/1 -> Battery Constraint/1(EMPwrElecVec)
  EM Constraint Front/2(InfeasibleEMVec) -> Infeasible conditions/1, Constraint Penalty Factor2/1  "InfeasibleEMF"
  Battery Constraint/2(BattCurr) -> BattCurr/1
  EM Constraint Front/1(WhlEMTrqSatVec) -> Add/1, [WhlEMTrqSatVecFrnt], WhlEMTrqSatVecFrnt/1
  WhlTrqCmd/1 -> Wheel Torque Vector Logic/1(WhlTrqCmd), Add1/1, EM Constraint Rear/1(WhlTrqCmd), EM Constraint Front/1(WhlTrqCmd)  "WhlTrqCmd"
  BattVin/1 -> Battery Constraint/2(BattVin)
  Saturation1/1 -> Product/1
  Veh2WhlSpd/1 -> Saturation1/1  "WhlSpd"
  Abs/1 -> TracPwrErr/1
  EM Constraint Rear/2(InfeasibleEMVec) -> Infeasible conditions/2, Constraint Penalty Factor1/1  "InfeasibleEMR"
  Infeasible conditions/1 -> InfeasibleFlagVec/1
  Battery Constraint/1(InfeasibleBatt) -> Infeasible conditions/3, Constraint Penalty Factor/1  "InfeasibleBatt"
  Add1/1 -> Product/2
  Add/1 -> Add1/2
  EM Constraint Rear/1(WhlEMTrqSatVec) -> [WhlEMTrqSatVecRear], Add/2, WhlEMTrqSatVecRear/1

== system EvPowertrainController2EM_r3/Torque Vectoring/No Torque Vectoring ==
  EMTrqCmd : Inport
  EMTrqCmdFinal : Outport  VectorParamsAs1DForOutWhenUnconnected=off
  wires:
  EMTrqCmd/1 -> EMTrqCmdFinal/1

== system EvPowertrainController2EM_r3/Accel Pedal to Traction Wheel Torque Request/EM2WhlTrq/2EM ==
  note: Use VehSpd instead of EMSpd or
      | WhlSpd in case wheel or EM are
      | undergoing slipping / have oscillations.
  note: Reflect EMTrq to WhlTrq
      | due to possible gearing
      | differences
  Gear : Inport
  VehSpd : Inport  Port=2
  Add : Sum
  EMTrq2WhlTrqFrnt : Subsystem  Variant=on  VariantControlMode=label  VariantControl=1  LabelModeActiveChoice=3
  EMTrq2WhlTrqRear : Subsystem  Variant=on  VariantControlMode=label  VariantControl=1  LabelModeActiveChoice=3
  Maximum Torque Front Axle : Subsystem
  Maximum Torque Rear Axle : Subsystem
  VehSpd2EMSpd : Subsystem  Variant=on  VariantControlMode=label  VariantControl=1  LabelModeActiveChoice=3
  WhlTrqCmd : Outport
  wires:
  VehSpd2EMSpd/2(EMSpdRearAxl) -> Maximum Torque Rear Axle/1(EMSpd), EMTrq2WhlTrqRear/3(EMSpd)
  EMTrq2WhlTrqRear/1(WhlMotTrq) -> Add/2
  Add/1 -> WhlTrqCmd/1
  VehSpd/1 -> VehSpd2EMSpd/2(VehSpd)
  EMTrq2WhlTrqFrnt/1(WhlMotTrq) -> Add/1
  Gear/1 -> EMTrq2WhlTrqRear/1(Gear), EMTrq2WhlTrqFrnt/1(Gear), VehSpd2EMSpd/1(Gear)
  Maximum Torque Rear Axle/1(EMTrq) -> EMTrq2WhlTrqRear/2(EMTrqCmd)
  VehSpd2EMSpd/1(EMSpdFrntAxl) -> Maximum Torque Front Axle/1(EMSpd), EMTrq2WhlTrqFrnt/3(EMSpd)
  Maximum Torque Front Axle/1(EMTrq) -> EMTrq2WhlTrqFrnt/2(EMTrqCmd)

== system EvPowertrainController2EM_r3/Accel Pedal to Traction Wheel Torque Request/EM2WhlTrq/3EM Dual Front ==
  note: Reflect EMTrq to WhlTrq
      | due to possible gearing
      | differences
  note: Use VehSpd instead of EMSpd or
      | WhlSpd in case wheel or EM are
      | undergoing slipping / have oscillations.
  Gear : Inport
  VehSpd : Inport  Port=2
  Add : Sum
  EMTrq2WhlTrqFrnt : Subsystem  Variant=on  VariantControlMode=label  VariantControl=1  LabelModeActiveChoice=3
  EMTrq2WhlTrqRear : Subsystem  Variant=on  VariantControlMode=label  VariantControl=1  LabelModeActiveChoice=3
  Maximum Torque Front Axle : Subsystem
  Maximum Torque Rear Axle : Subsystem
  VehSpd2EMSpd : Subsystem  Variant=on  VariantControlMode=label  VariantControl=1  LabelModeActiveChoice=3
  WhlTrqCmd : Outport
  wires:
  Maximum Torque Front Axle/1(EMTrq) -> EMTrq2WhlTrqFrnt/2(EMTrqCmd)
  VehSpd2EMSpd/1(EMSpdFrntAxl) -> EMTrq2WhlTrqFrnt/3(EMSpd), Maximum Torque Front Axle/1(EMSpd)
  Maximum Torque Rear Axle/1(EMTrq) -> EMTrq2WhlTrqRear/2(EMTrqCmd)
  Gear/1 -> VehSpd2EMSpd/1(Gear), EMTrq2WhlTrqFrnt/1(Gear), EMTrq2WhlTrqRear/1(Gear)
  EMTrq2WhlTrqFrnt/1(WhlMotTrq) -> Add/1
  VehSpd/1 -> VehSpd2EMSpd/2(VehSpd)
  Add/1 -> WhlTrqCmd/1
  EMTrq2WhlTrqRear/1(WhlMotTrq) -> Add/2
  VehSpd2EMSpd/2(EMSpdRearAxl) -> EMTrq2WhlTrqRear/3(EMSpd), Maximum Torque Rear Axle/1(EMSpd)

== system EvPowertrainController2EM_r3/Accel Pedal to Traction Wheel Torque Request/EM2WhlTrq/3EM Dual Rear ==
  note: Use VehSpd instead of EMSpd or
      | WhlSpd in case wheel or EM are
      | undergoing slipping / have oscillations.
  note: Reflect EMTrq to WhlTrq
      | due to possible gearing
      | differences
  Gear : Inport
  VehSpd : Inport  Port=2
  Add : Sum
  EMTrq2WhlTrqFrnt : Subsystem  Variant=on  VariantControlMode=label  VariantControl=1  LabelModeActiveChoice=3
  EMTrq2WhlTrqRear : Subsystem  Variant=on  VariantControlMode=label  VariantControl=1  LabelModeActiveChoice=3
  Maximum Torque Front Axle : Subsystem
  Maximum Torque Rear Axle : Subsystem
  VehSpd2EMSpd : Subsystem  Variant=on  VariantControlMode=label  VariantControl=1  LabelModeActiveChoice=3
  WhlTrqCmd : Outport
  wires:
  VehSpd2EMSpd/2(EMSpdRearAxl) -> Maximum Torque Rear Axle/1(EMSpd), EMTrq2WhlTrqRear/3(EMSpd)
  EMTrq2WhlTrqRear/1(WhlMotTrq) -> Add/2
  Add/1 -> WhlTrqCmd/1
  VehSpd/1 -> VehSpd2EMSpd/2(VehSpd)
  EMTrq2WhlTrqFrnt/1(WhlMotTrq) -> Add/1
  Gear/1 -> EMTrq2WhlTrqRear/1(Gear), EMTrq2WhlTrqFrnt/1(Gear), VehSpd2EMSpd/1(Gear)
  Maximum Torque Rear Axle/1(EMTrq) -> EMTrq2WhlTrqRear/2(EMTrqCmd)
  VehSpd2EMSpd/1(EMSpdFrntAxl) -> Maximum Torque Front Axle/1(EMSpd), EMTrq2WhlTrqFrnt/3(EMSpd)
  Maximum Torque Front Axle/1(EMTrq) -> EMTrq2WhlTrqFrnt/2(EMTrqCmd)

== system EvPowertrainController2EM_r3/Accel Pedal to Traction Wheel Torque Request/EM2WhlTrq/4EM ==
  note: Reflect EMTrq to WhlTrq
      | due to possible gearing
      | differences
  note: Use VehSpd instead of EMSpd or
      | WhlSpd in case wheel or EM are
      | undergoing slipping / have oscillations.
  Gear : Inport
  VehSpd : Inport  Port=2
  Add : Sum
  EMTrq2WhlTrqFrnt : Subsystem  Variant=on  VariantControlMode=label  VariantControl=1  LabelModeActiveChoice=3
  EMTrq2WhlTrqRear : Subsystem  Variant=on  VariantControlMode=label  VariantControl=1  LabelModeActiveChoice=3
  Maximum Torque Front Axle : Subsystem
  Maximum Torque Rear Axle : Subsystem
  VehSpd2EMSpd : Subsystem  Variant=on  VariantControlMode=label  VariantControl=1  LabelModeActiveChoice=3
  WhlTrqCmd : Outport
  wires:
  Maximum Torque Front Axle/1(EMTrq) -> EMTrq2WhlTrqFrnt/2(EMTrqCmd)
  VehSpd2EMSpd/1(EMSpdFrntAxl) -> EMTrq2WhlTrqFrnt/3(EMSpd), Maximum Torque Front Axle/1(EMSpd)
  Maximum Torque Rear Axle/1(EMTrq) -> EMTrq2WhlTrqRear/2(EMTrqCmd)
  Gear/1 -> VehSpd2EMSpd/1(Gear), EMTrq2WhlTrqFrnt/1(Gear), EMTrq2WhlTrqRear/1(Gear)
  EMTrq2WhlTrqFrnt/1(WhlMotTrq) -> Add/1
  VehSpd/1 -> VehSpd2EMSpd/2(VehSpd)
  Add/1 -> WhlTrqCmd/1
  EMTrq2WhlTrqRear/1(WhlMotTrq) -> Add/2
  VehSpd2EMSpd/2(EMSpdRearAxl) -> EMTrq2WhlTrqRear/3(EMSpd), Maximum Torque Rear Axle/1(EMSpd)

== system EvPowertrainController2EM_r3/Energy Management/Calculate Average EMSpd and Wheel Torque Curves for Front and Rear Axles/2EM ==
  note: Reflect EMTrq to WhlTrq
      | due to possible gearing
      | differences
  EMSpd : Inport
  Gear : Inport  Port=2
  EMTrq2WhlTrqFrnt : Subsystem  Variant=on  VariantControlMode=label  VariantControl=1  LabelModeActiveChoice=3
  EMTrq2WhlTrqRear : Subsystem  Variant=on  VariantControlMode=label  VariantControl=1  LabelModeActiveChoice=3
  Maximum Torque Front Axle : Subsystem
  Maximum Torque Rear Axle : Subsystem
  Selector : Selector  InputPortWidth=2  IndexOptions=Index vector (dialog)  Indices=[1]  OutputSizes=1
  Selector1 : Selector  InputPortWidth=2  IndexOptions=Index vector (dialog)  Indices=[2]  OutputSizes=1
  Vector Concatenate : Concatenate
  Vector Concatenate1 : Concatenate
  EMAvgSpdVec : Outport
  WhlTrqMaxVec : Outport  Port=2
  wires:
  Vector Concatenate1/1 -> EMAvgSpdVec/1
  Vector Concatenate/1 -> WhlTrqMaxVec/1
  Maximum Torque Front Axle/1(EMTrq) -> EMTrq2WhlTrqFrnt/2(EMTrqCmd)
  Maximum Torque Rear Axle/1(EMTrq) -> EMTrq2WhlTrqRear/2(EMTrqCmd)
  EMTrq2WhlTrqFrnt/1(WhlMotTrq) -> Vector Concatenate/1
  Selector/1 -> Maximum Torque Front Axle/1(EMSpd), EMTrq2WhlTrqFrnt/3(EMSpd), Vector Concatenate1/1
  Gear/1 -> EMTrq2WhlTrqRear/1(Gear), EMTrq2WhlTrqFrnt/1(Gear)
  EMTrq2WhlTrqRear/1(WhlMotTrq) -> Vector Concatenate/2
  Selector1/1 -> Maximum Torque Rear Axle/1(EMSpd), EMTrq2WhlTrqRear/3(EMSpd), Vector Concatenate1/2
  EMSpd/1 -> Selector1/1, Selector/1

== system EvPowertrainController2EM_r3/Energy Management/Calculate Average EMSpd and Wheel Torque Curves for Front and Rear Axles/3EM Dual Front ==
  note: Reflect EMTrq to WhlTrq
      | due to possible gearing
      | differences
  note: Calculate average speed
      | of EMs on axle
  EMSpd : Inport
  Gear : Inport  Port=2
  EMTrq2WhlTrqFrnt : Subsystem  Variant=on  VariantControlMode=label  VariantControl=1  LabelModeActiveChoice=3
  EMTrq2WhlTrqRear : Subsystem  Variant=on  VariantControlMode=label  VariantControl=1  LabelModeActiveChoice=3
  Gain : Gain  Gain=1/2
  Maximum Torque Front Axle : Subsystem
  Maximum Torque Rear Axle : Subsystem
  Selector : Selector  InputPortWidth=3  IndexOptions=Index vector (dialog)  Indices=[1 2]  OutputSizes=1
  Selector1 : Selector  InputPortWidth=3  IndexOptions=Index vector (dialog)  Indices=[3]  OutputSizes=1
  Sum of Elements : Sum  Inputs=+
  Vector Concatenate : Concatenate
  Vector Concatenate1 : Concatenate
  EMAvgSpdVec : Outport
  WhlTrqMaxVec : Outport  Port=2
  wires:
  Vector Concatenate1/1 -> EMAvgSpdVec/1
  Vector Concatenate/1 -> WhlTrqMaxVec/1
  EMTrq2WhlTrqFrnt/1(WhlMotTrq) -> Vector Concatenate/1
  EMTrq2WhlTrqRear/1(WhlMotTrq) -> Vector Concatenate/2
  Selector1/1 -> Vector Concatenate1/2, EMTrq2WhlTrqRear/3(EMSpd), Maximum Torque Rear Axle/1(EMSpd)
  Gear/1 -> EMTrq2WhlTrqFrnt/1(Gear), EMTrq2WhlTrqRear/1(Gear)
  Gain/1 -> Maximum Torque Front Axle/1(EMSpd), EMTrq2WhlTrqFrnt/3(EMSpd), Vector Concatenate1/1
  Maximum Torque Front Axle/1(EMTrq) -> EMTrq2WhlTrqFrnt/2(EMTrqCmd)
  Maximum Torque Rear Axle/1(EMTrq) -> EMTrq2WhlTrqRear/2(EMTrqCmd)
  Sum of Elements/1 -> Gain/1
  EMSpd/1 -> Selector/1, Selector1/1
  Selector/1 -> Sum of Elements/1

== system EvPowertrainController2EM_r3/Energy Management/Calculate Average EMSpd and Wheel Torque Curves for Front and Rear Axles/3EM Dual Rear ==
  note: Reflect EMTrq to WhlTrq
      | due to possible gearing
      | differences
  note: Calculate average speed
      | of EMs on axle
  EMSpd : Inport
  Gear : Inport  Port=2
  EMTrq2WhlTrqFrnt : Subsystem  Variant=on  VariantControlMode=label  VariantControl=1  LabelModeActiveChoice=3
  EMTrq2WhlTrqRear : Subsystem  Variant=on  VariantControlMode=label  VariantControl=1  LabelModeActiveChoice=3
  Gain : Gain  Gain=1/2
  Maximum Torque Front Axle : Subsystem
  Maximum Torque Rear Axle : Subsystem
  Selector : Selector  InputPortWidth=3  IndexOptions=Index vector (dialog)  Indices=[2 3]  OutputSizes=1
  Selector1 : Selector  InputPortWidth=3  IndexOptions=Index vector (dialog)  Indices=[1]  OutputSizes=1
  Sum of Elements : Sum  Inputs=+
  Vector Concatenate : Concatenate
  Vector Concatenate1 : Concatenate
  EMAvgSpdVec : Outport
  WhlTrqMaxVec : Outport  Port=2
  wires:
  Vector Concatenate1/1 -> EMAvgSpdVec/1
  Vector Concatenate/1 -> WhlTrqMaxVec/1
  EMTrq2WhlTrqFrnt/1(WhlMotTrq) -> Vector Concatenate/1
  Gear/1 -> EMTrq2WhlTrqRear/1(Gear), EMTrq2WhlTrqFrnt/1(Gear)
  Selector1/1 -> Maximum Torque Front Axle/1(EMSpd), EMTrq2WhlTrqFrnt/3(EMSpd), Vector Concatenate1/1
  Maximum Torque Front Axle/1(EMTrq) -> EMTrq2WhlTrqFrnt/2(EMTrqCmd)
  Maximum Torque Rear Axle/1(EMTrq) -> EMTrq2WhlTrqRear/2(EMTrqCmd)
  Gain/1 -> Maximum Torque Rear Axle/1(EMSpd), EMTrq2WhlTrqRear/3(EMSpd), Vector Concatenate1/2
  EMTrq2WhlTrqRear/1(WhlMotTrq) -> Vector Concatenate/2
  Selector/1 -> Sum of Elements/1
  EMSpd/1 -> Selector/1, Selector1/1
  Sum of Elements/1 -> Gain/1

== system EvPowertrainController2EM_r3/Energy Management/Calculate Average EMSpd and Wheel Torque Curves for Front and Rear Axles/4EM ==
  note: Reflect EMTrq to WhlTrq
      | due to possible gearing
      | differences
  note: Calculate average speed
      | of EMs on axle
  EMSpd : Inport
  Gear : Inport  Port=2
  EMTrq2WhlTrqFrnt : Subsystem  Variant=on  VariantControlMode=label  VariantControl=1  LabelModeActiveChoice=3
  EMTrq2WhlTrqRear : Subsystem  Variant=on  VariantControlMode=label  VariantControl=1  LabelModeActiveChoice=3
  Gain : Gain  Gain=1/2
  Gain1 : Gain  Gain=1/2
  Maximum Torque Front Axle : Subsystem
  Maximum Torque Rear Axle : Subsystem
  Selector : Selector  InputPortWidth=4  IndexOptions=Index vector (dialog)  Indices=[3 4]  OutputSizes=1
  Selector1 : Selector  InputPortWidth=4  IndexOptions=Index vector (dialog)  Indices=[1 2]  OutputSizes=1
  Sum of Elements : Sum  Inputs=+
  Sum of Elements1 : Sum  Inputs=+
  Vector Concatenate : Concatenate
  Vector Concatenate1 : Concatenate
  EMAvgSpdVec : Outport
  WhlTrqMaxVec : Outport  Port=2
  wires:
  Vector Concatenate1/1 -> EMAvgSpdVec/1
  Vector Concatenate/1 -> WhlTrqMaxVec/1
  Gain/1 -> EMTrq2WhlTrqRear/3(EMSpd), Maximum Torque Rear Axle/1(EMSpd), Vector Concatenate1/2
  Gear/1 -> EMTrq2WhlTrqFrnt/1(Gear), EMTrq2WhlTrqRear/1(Gear)
  EMTrq2WhlTrqFrnt/1(WhlMotTrq) -> Vector Concatenate/1
  Gain1/1 -> Maximum Torque Front Axle/1(EMSpd), EMTrq2WhlTrqFrnt/3(EMSpd), Vector Concatenate1/1
  Maximum Torque Rear Axle/1(EMTrq) -> EMTrq2WhlTrqRear/2(EMTrqCmd)
  Maximum Torque Front Axle/1(EMTrq) -> EMTrq2WhlTrqFrnt/2(EMTrqCmd)
  EMTrq2WhlTrqRear/1(WhlMotTrq) -> Vector Concatenate/2
  Sum of Elements1/1 -> Gain1/1
  Sum of Elements/1 -> Gain/1
  EMSpd/1 -> Selector1/1, Selector/1
  Selector1/1 -> Sum of Elements1/1
  Selector/1 -> Sum of Elements/1

== system EvPowertrainController2EM_r3/Energy Management/Control Domain /Front Axle EM Torque Vector ==
  EMAvgSpdVec : Inport
  2EM or 3EM Dual Rear : Subsystem  VariantControl=2EM or 3EM Dual Rear
  3EM Dual Front or 4EM : Subsystem  VariantControl=3EM Dual Front or 4EM
  WhlEMFrntVecPos : Outport
  WhlEMFrntVecNeg : Outport  Port=2

== system EvPowertrainController2EM_r3/Energy Management/Control Domain /Rear Axle EM Torque Vector ==
  EMAvgSpdVec : Inport
  2EM or 3EM Dual Front : Subsystem  VariantControl=2EM or 3EM Dual Front
  3EM Dual Rear or 4EM : Subsystem  VariantControl=3EM Dual Rear or 4EM
  WhlEMRearVecPos : Outport
  WhlEMRearVecNeg : Outport  Port=2

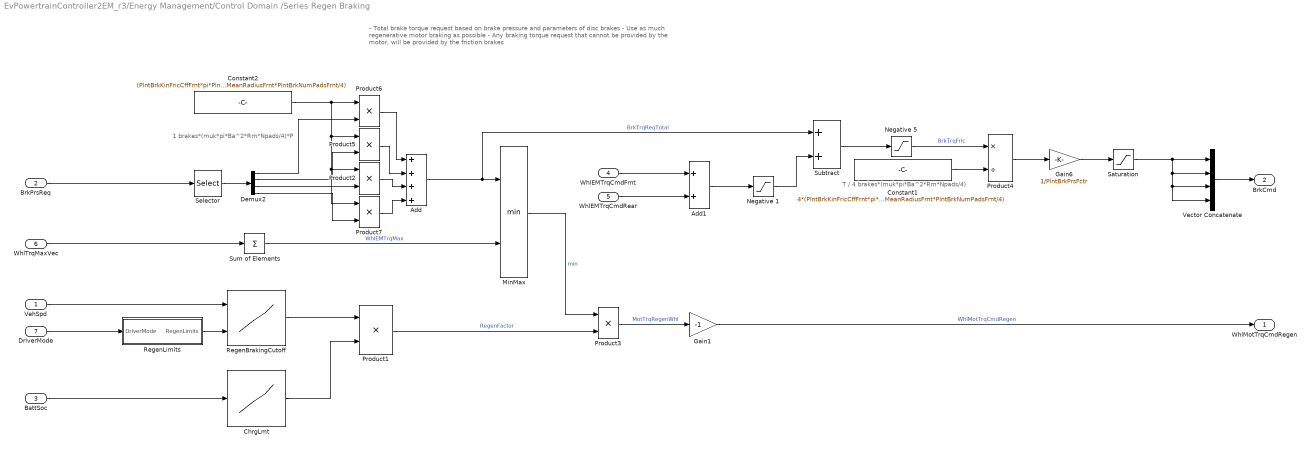
== system EvPowertrainController2EM_r3/Energy Management/Control Domain /Series Regen Braking ==
  note: 1 brakes*(muk*pi*Ba^2*Rm*Npads/4)*P
  note: T / 4 brakes*(muk*pi*Ba^2*Rm*Npads/4)
  note: - Total brake torque request based on brake pressure and parameters of disc brakes
      | - Use as much regenerative motor braking as possible
      | - Any braking torque request that cannot be provided by the motor, will be provided by the friction brakes
  VehSpd : Inport
  "BrkPrsReq " : Inport  Port=2
  BattSoc : Inport  Port=3
  WhlEMTrqCmdFrnt : Inport  Port=4
  WhlEMTrqCmdRear : Inport  Port=5
  WhlTrqMaxVec : Inport  Port=6
  DriverMode : Inport  Port=7
  Add : Sum  Inputs=++++
  Add1 : Sum
  ChrgLmt : Lookup_n-D  NumberOfTableDimensions=1  BreakpointsForDimension1=CtrlVcuEvSocBpt  Table=CtrlVcuEvChrgLmtBpt  ExtrapMethod=Clip  UseLastTableValue=on  InternalRulePriority=Speed  RndMeth=Simplest
  Constant1 : Constant  Value=4*(PlntBrkKinFricCffFrnt*pi*PlntBrkActrBoreFrnt^2*PlntBrkPadMeanRadiusFrnt*PlntBrkNumPadsFrnt/4)
  Constant2 : Constant  Value=(PlntBrkKinFricCffFrnt*pi*PlntBrkActrBoreFrnt^2*PlntBrkPadMeanRadiusFrnt*PlntBrkNumPadsFrnt/4)
  Demux2 : Demux
  Gain1 : Gain  Gain=-1
  Gain6 : Gain  Gain=1/PlntBrkPrsFctr
  MinMax : MinMax  Inputs=2
  Negative 1 : Saturate  UpperLimit=0  LowerLimit=-inf
  Negative 5 : Saturate  UpperLimit=inf  LowerLimit=0
  Product{1..3,5..7} (6 alike) : Product
  Product4 : Product  Inputs=*/
  RegenBrakingCutoff : Lookup_n-D  NumberOfTableDimensions=1  BreakpointsForDimension1Source=Input port  BreakpointsForDimension1=CtrlVcuEvRegenBrkSpdBpt  Table=CtrlVcuEvRegenBrkCutOff  ExtrapMethod=Clip  UseLastTableValue=on  InternalRulePriority=Speed  RndMeth=Simplest
      settings: InputPortMap=u0,p5
  RegenLimits : Subsystem
  Saturation : Saturate  UpperLimit=1  LowerLimit=0
  Selector : Selector  InputPortWidth=4  IndexOptions=Index vector (dialog)  Indices=[1 2 3 4]  OutputSizes=1
  Subtract : Sum
  Sum of Elements : Sum  Inputs=+
  Vector Concatenate : Concatenate  NumInputs=4
  " WhlMotTrqCmdRegen" : Outport  VectorParamsAs1DForOutWhenUnconnected=off
  " BrkCmd" : Outport  Port=2  VectorParamsAs1DForOutWhenUnconnected=off
  wires:
  DriverMode/1 -> RegenLimits/1(DriverMode)
  RegenLimits/1(RegenLimits) -> RegenBrakingCutoff/2
  WhlEMTrqCmdRear/1 -> Add1/2
  WhlEMTrqCmdFrnt/1 -> Add1/1
  Constant2/1 -> Product6/1, Product5/1, Product2/1, Product7/1
  Demux2/4 -> Product7/2
  Demux2/3 -> Product2/2
  Product7/1 -> Add/4
  Product2/1 -> Add/3
  Negative 1/1 -> Subtract/2
  Add1/1 -> Negative 1/1
  Product3/1 -> Gain1/1  "MotTrqRegenWhl"
  Gain1/1 -> " WhlMotTrqCmdRegen"/1  "WhlMotTrqCmdRegen"
  WhlTrqMaxVec/1 -> Sum of Elements/1
  Saturation/1 -> Vector Concatenate/1, Vector Concatenate/2, Vector Concatenate/4, Vector Concatenate/3
  Product4/1 -> Gain6/1
  Gain6/1 -> Saturation/1
  Vector Concatenate/1 -> " BrkCmd"/1
  "BrkPrsReq "/1 -> Selector/1
  Add/1 -> MinMax/1, Subtract/1  "BrkTrqReqTotal"
  Product5/1 -> Add/2
  Product6/1 -> Add/1
  Selector/1 -> Demux2/1
  Demux2/1 -> Product6/2
  Demux2/2 -> Product5/2
  Sum of Elements/1 -> MinMax/2  "WhlEMTrqMax"
  Negative 5/1 -> Product4/1  "BrkTrqFric"
  BattSoc/1 -> ChrgLmt/1
  Subtract/1 -> Negative 5/1
  Product1/1 -> Product3/2  "RegenFactor"
  RegenBrakingCutoff/1 -> Product1/1
  VehSpd/1 -> RegenBrakingCutoff/1
  ChrgLmt/1 -> Product1/2
  MinMax/1 -> Product3/1  "min"
  Constant1/1 -> Product4/2

== system EvPowertrainController2EM_r3/Energy Management/Convert Whl to EMTrq Vector/2EM ==
  WhlEMTrqCmdFrnt : Inport
  WhlEMTrqCmdRear : Inport  Port=2
  EMAvgSpdVec : Inport  Port=3
  Diff Eta : Subsystem
  Diff Eta1 : Subsystem
  Divide1 : Product  Inputs=/*
  Divide2 : Product  Inputs=/*
  Gain1 : Gain  Gain=1/PlntDiffrntl2Ratio
  Gain3 : Gain  Gain=1/PlntDiffrntlRatio
  Selector : Selector  InputPortWidth=2  IndexOptions=Index vector (dialog)  Indices=[1]  OutputSizes=1
  Selector1 : Selector  InputPortWidth=2  IndexOptions=Index vector (dialog)  Indices=[2]  OutputSizes=1
  Unit Delay : UnitDelay  SampleTime=-1  HasFrameUpgradeWarning=on
  Unit Delay1 : UnitDelay  SampleTime=-1  HasFrameUpgradeWarning=on
  Vector Concatenate1 : Concatenate
  EMTrqCmd : Outport
  wires:
  Vector Concatenate1/1 -> EMTrqCmd/1
  Selector1/1 -> Diff Eta1/1(SpdIn)
  EMAvgSpdVec/1 -> Selector/1, Selector1/1
  Gain1/1 -> Divide1/2
  Divide1/1 -> Vector Concatenate1/2, Unit Delay1/1
  Unit Delay1/1 -> Diff Eta1/2(TrqIn)
  Diff Eta1/1(eta) -> Divide1/1
  Diff Eta/1(eta) -> Divide2/1
  Unit Delay/1 -> Diff Eta/2(TrqIn)
  Selector/1 -> Diff Eta/1(SpdIn)
  WhlEMTrqCmdFrnt/1 -> Gain3/1
  Divide2/1 -> Unit Delay/1, Vector Concatenate1/1
  Gain3/1 -> Divide2/2
  WhlEMTrqCmdRear/1 -> Gain1/1

== system EvPowertrainController2EM_r3/Energy Management/Convert Whl to EMTrq Vector/3EM Dual Front ==
  WhlEMTrqCmdFrnt : Inport
  WhlEMTrqCmdRear : Inport  Port=2
  EMAvgSpdVec : Inport  Port=3
  Diff Eta : Subsystem
  Divide1 : Product  Inputs=/*
  Divide2 : Product  Inputs=/*
  Dual EMs : Gain  Gain=1/2
  Gain1 : Gain  Gain=1/PlntDiffrntl2Ratio
  Gain3 : Gain  Gain=1/PlntEMWhlGearRatioFL
  Gear Eta : Subsystem
  Selector : Selector  InputPortWidth=2  IndexOptions=Index vector (dialog)  Indices=[1]  OutputSizes=1
  Selector1 : Selector  InputPortWidth=2  IndexOptions=Index vector (dialog)  Indices=[2]  OutputSizes=1
  Unit Delay : UnitDelay  SampleTime=-1  HasFrameUpgradeWarning=on
  Unit Delay1 : UnitDelay  SampleTime=-1  HasFrameUpgradeWarning=on
  Vector Concatenate : Concatenate  NumInputs=3
  EMTrqCmd : Outport
  wires:
  Dual EMs/1 -> Gain3/1
  Divide2/1 -> Unit Delay/1, Vector Concatenate/2, Vector Concatenate/1
  Vector Concatenate/1 -> EMTrqCmd/1
  Divide1/1 -> Unit Delay1/1, Vector Concatenate/3
  WhlEMTrqCmdRear/1 -> Gain1/1
  Gain3/1 -> Divide2/2
  WhlEMTrqCmdFrnt/1 -> Dual EMs/1
  Selector/1 -> Gear Eta/1(SpdIn)
  Unit Delay/1 -> Gear Eta/2(TrqIn)
  Gear Eta/1(eta) -> Divide2/1
  Diff Eta/1(eta) -> Divide1/1
  Unit Delay1/1 -> Diff Eta/2(TrqIn)
  Gain1/1 -> Divide1/2
  EMAvgSpdVec/1 -> Selector1/1, Selector/1
  Selector1/1 -> Diff Eta/1(SpdIn)

== system EvPowertrainController2EM_r3/Energy Management/Convert Whl to EMTrq Vector/3EM Dual Rear ==
  WhlEMTrqCmdFrnt : Inport
  WhlEMTrqCmdRear : Inport  Port=2
  EMAvgSpdVec : Inport  Port=3
  Diff Eta : Subsystem
  Divide1 : Product  Inputs=/*
  Divide2 : Product  Inputs=/*
  Dual EMs : Gain  Gain=1/2
  Gain1 : Gain  Gain=1/PlntEMWhlGearRatioRL
  Gain3 : Gain  Gain=1/PlntDiffrntlRatio
  Gear Eta : Subsystem
  Selector : Selector  InputPortWidth=2  IndexOptions=Index vector (dialog)  Indices=[1]  OutputSizes=1
  Selector1 : Selector  InputPortWidth=2  IndexOptions=Index vector (dialog)  Indices=[2]  OutputSizes=1
  Unit Delay : UnitDelay  SampleTime=-1  HasFrameUpgradeWarning=on
  Unit Delay1 : UnitDelay  SampleTime=-1  HasFrameUpgradeWarning=on
  Vector Concatenate : Concatenate  NumInputs=3
  EMTrqCmd : Outport
  wires:
  Dual EMs/1 -> Gain1/1
  Selector1/1 -> Gear Eta/1(SpdIn)
  EMAvgSpdVec/1 -> Selector/1, Selector1/1
  Gain1/1 -> Divide1/2
  Unit Delay1/1 -> Gear Eta/2(TrqIn)
  Gear Eta/1(eta) -> Divide1/1
  Diff Eta/1(eta) -> Divide2/1
  Unit Delay/1 -> Diff Eta/2(TrqIn)
  Selector/1 -> Diff Eta/1(SpdIn)
  Gain3/1 -> Divide2/2
  WhlEMTrqCmdRear/1 -> Dual EMs/1
  Divide1/1 -> Vector Concatenate/3, Vector Concatenate/2, Unit Delay1/1
  Vector Concatenate/1 -> EMTrqCmd/1
  Divide2/1 -> Vector Concatenate/1, Unit Delay/1
  WhlEMTrqCmdFrnt/1 -> Gain3/1

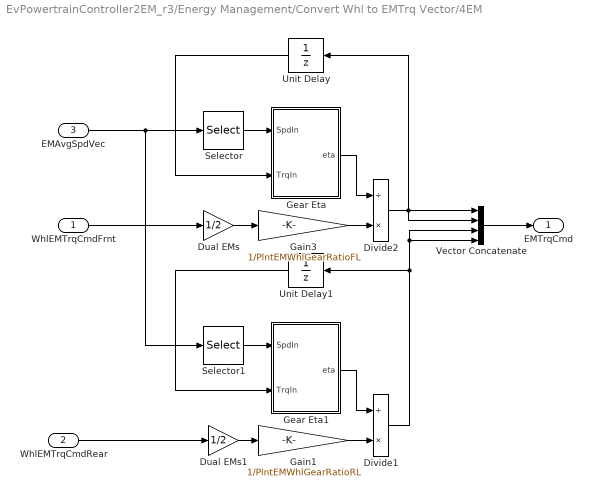
== system EvPowertrainController2EM_r3/Energy Management/Convert Whl to EMTrq Vector/4EM ==
  WhlEMTrqCmdFrnt : Inport
  WhlEMTrqCmdRear : Inport  Port=2
  EMAvgSpdVec : Inport  Port=3
  Divide1 : Product  Inputs=/*
  Divide2 : Product  Inputs=/*
  Dual EMs : Gain  Gain=1/2
  Dual EMs1 : Gain  Gain=1/2
  Gain1 : Gain  Gain=1/PlntEMWhlGearRatioRL
  Gain3 : Gain  Gain=1/PlntEMWhlGearRatioFL
  Gear Eta : Subsystem
  Gear Eta1 : Subsystem
  Selector : Selector  InputPortWidth=2  IndexOptions=Index vector (dialog)  Indices=[1]  OutputSizes=1
  Selector1 : Selector  InputPortWidth=2  IndexOptions=Index vector (dialog)  Indices=[2]  OutputSizes=1
  Unit Delay : UnitDelay  SampleTime=-1  HasFrameUpgradeWarning=on
  Unit Delay1 : UnitDelay  SampleTime=-1  HasFrameUpgradeWarning=on
  Vector Concatenate : Concatenate  NumInputs=4
  EMTrqCmd : Outport
  wires:
  Dual EMs/1 -> Gain3/1
  WhlEMTrqCmdFrnt/1 -> Dual EMs/1
  Divide2/1 -> Vector Concatenate/1, Unit Delay/1, Vector Concatenate/2
  Vector Concatenate/1 -> EMTrqCmd/1
  Divide1/1 -> Unit Delay1/1, Vector Concatenate/3, Vector Concatenate/4
  WhlEMTrqCmdRear/1 -> Dual EMs1/1
  Gain3/1 -> Divide2/2
  Selector/1 -> Gear Eta/1(SpdIn)
  Unit Delay/1 -> Gear Eta/2(TrqIn)
  Gear Eta/1(eta) -> Divide2/1
  Gear Eta1/1(eta) -> Divide1/1
  Unit Delay1/1 -> Gear Eta1/2(TrqIn)
  Gain1/1 -> Divide1/2
  EMAvgSpdVec/1 -> Selector1/1, Selector/1
  Selector1/1 -> Gear Eta1/1(SpdIn)
  Dual EMs1/1 -> Gain1/1

== system EvPowertrainController2EM_r3/Energy Management/Hamiltonian computation and minimization/Pwr Rate Limit ==
  note: Alternative to using
      | abs funciton
  note: There could be instances where an mot trq command produces the minimum cost, but differs greatly from the previously selected mot trq.
      |
      | This function will calculate the difference in power between the current mot power vector and the previously selected mot pwr.  This term is added to the total cost function, and will help limit the rate at which the mot power (and torque) can change from time step to time step.
  note: This table helps reduce rapid oscillations in torque
      | that can occur when operating at WOT conditions which
      | can result in the torque being limited by the BMS.
  WhlEMTrqVec : Inport
  WhlSpd : Inport  Port=2
  PrevWhlEMTrqCmd : Inport  Port=3
  AccelPdl : Inport  Port=4
  1-D Lookup Table : Lookup_n-D  NumberOfTableDimensions=1  BreakpointsForDimension1=CtrlVcuAccelPdlBpts  BeginIndexSearchUsingPreviousIndexResult=on  Table=CtrlVcuPwrRatePnlty  ExtrapMethod=Clip  UseLastTableValue=on  InternalRulePriority=Speed  RndMeth=Simplest
  Product{,1,6..7} (4 alike) : Product
  Sqrt1 : Sqrt
  Subtract : Sum  Inputs=+-
  W2kW : Gain  Gain=1/1000
  EMPwrDelta : Outport  VectorParamsAs1DForOutWhenUnconnected=off
  wires:
  1-D Lookup Table/1 -> Product/2
  AccelPdl/1 -> 1-D Lookup Table/1
  Product/1 -> EMPwrDelta/1
  W2kW/1 -> Product/1
  WhlEMTrqVec/1 -> Product6/1
  Sqrt1/1 -> W2kW/1
  Subtract/1 -> Product7/2, Product7/1
  PrevWhlEMTrqCmd/1 -> Product1/2
  WhlSpd/1 -> Product1/1, Product6/2
  Product1/1 -> Subtract/2  "PrevPwr"
  Product6/1 -> Subtract/1  "PwrVec"
  Product7/1 -> Sqrt1/1
